simulink model "model_2"  (R2014b)
settings: Solver=ode45  StartTime=0.0  StopTime=10.0  RelTol=1e-3
settings Model: Creator=Shane Reynolds  LastModifiedBy=Shane Reynolds

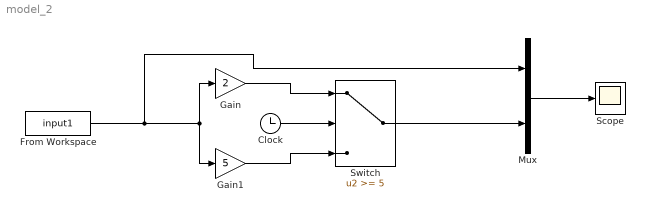
== system model_2 ==
  Clock : Clock
  From Workspace : FromWorkspace  VariableName=input1  SampleTime=0
  Gain : Gain  Gain=2
  Gain1 : Gain  Gain=5
  Mux : Mux  Inputs=2
  Scope : Scope
  Switch : Switch  Threshold=5
  wires:
  Mux/1 -> Scope/1
  From Workspace/1 -> Mux/1, Gain1/1, Gain/1
  Clock/1 -> Switch/2
  Gain/1 -> Switch/1
  Gain1/1 -> Switch/3
  Switch/1 -> Mux/2
